simulink model "rtwdemo_voidvoidfcn"  (Simulink 7.1)
settings: Solver=FixedStepDiscrete  StartTime=0.0  StopTime=10.0  RelTol=1e-3
settings Model: Creator=ajayaram  LastModifiedBy=ajayaram
settings SolverCC: AutoInsertRateTranBlk=on
settings DataIOCC: SaveOutput=off  SaveTime=off
settings OptimizationCC: InlineParams=on  InlineInvariantSignals=on  EnforceIntegerDowncast=off  StateBitsets=on  DataBitsets=on  UseTempVars=on  OptimizeModelRefInitCode=on  LifeSpan=1
settings RTWCC: SystemTargetFile=ert.tlc  GenCodeOnly=on  GenerateMakefile=off  TemplateMakefile=ert_default_tmf  Description=Real-Time Workshop Embedded Coder (no auto configuration)  GenerateReport=on  RTWVerbose=off  ProcessScript=ert_make_rtw_hook  IncludeHyperlinkInReport=on  LaunchReport=on
settings CodeAppCC: IgnoreCustomStorageClasses=off  CustomSymbolStrGlobalVar=rt$N$M  CustomSymbolStrType=$N$M  CustomSymbolStrFcn=$N$M$F  CustomSymbolStrMacro=$N$M
settings ERTTargetCC: GenerateSampleERTMain=on  SuppressErrorStatus=on  SupportAbsoluteTime=off  SupportNonFinite=off  SupportComplex=off  InlinedParameterPlacement=NonHierarchical  RootIOFormat=Structure reference  ERTCustomFileTemplate=example_file_process.tlc

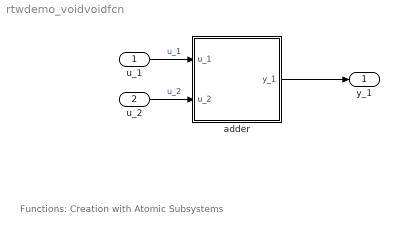
== system rtwdemo_voidvoidfcn ==
  note: Functions: Creation with Atomic Subsystems
  u_1 : Inport  OutDataType=sfix(16)  OutScaling=2^0
  u_2 : Inport  Port=2  OutDataType=sfix(16)  OutScaling=2^0
  adder : Subsystem  TreatAsAtomicUnit=on  RTWFcnName=adder  RTWFileName=adder
      settings: RTWSystemCode=Function  RTWFcnNameOpts=User specified  RTWFileNameOpts=User specified
  y_1 : Outport  OutDataType=sfix(16)  OutScaling=2^0
  wires:
  u_1/1 -> adder/1(u_1)  "u_1"
  adder/1(y_1) -> y_1/1
  u_2/1 -> adder/2(u_2)  "u_2"

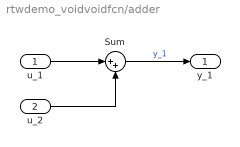
== system rtwdemo_voidvoidfcn/adder ==
  u_1 : Inport  OutDataType=sfix(16)  OutScaling=2^0
  u_2 : Inport  Port=2  OutDataType=sfix(16)  OutScaling=2^0
  Sum : Sum  Inputs=|++  OutDataType=sfix(16)  OutScaling=2^0
  y_1 : Outport  OutDataType=sfix(16)  OutScaling=2^0
  wires:
  u_1/1 -> Sum/1
  u_2/1 -> Sum/2
  Sum/1 -> y_1/1  "y_1"
